simulink model "oving2e"  (R2020b)
settings: Solver=VariableStepAuto  StartTime=0.0  StopTime=10.0  RelTol=1e-3
values from neighbouring files (symbols this model uses):
  K = 1    [oving2script.m]
  l = 1    [Oving2Var.mat]    (also in oving2script.m)
  T = 1    [Oving2Var.mat]    (also in oving2script.m)
  y_0 = 0    [oving2script.m]
undefined symbols (not defined in the file or in its folder): K_i, K_p, r_0
settings Model: Creator=crezl  LastModifiedBy=crezl

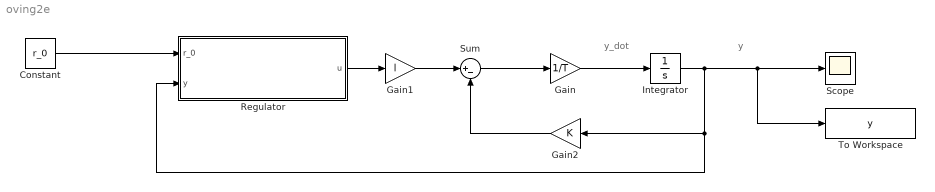
== system oving2e ==
  note: y_dot
  note: y
  Constant : Constant  Value=r_0
  Gain : Gain  Gain=1/T
  Gain1 : Gain  Gain=l
  Gain2 : Gain  Gain=K
  Integrator : Integrator  InitialCondition=y_0
  Regulator : Subsystem
  Scope : Scope
  Sum : Sum  Inputs=|+-
  To Workspace : ToWorkspace  VariableName=y  SaveFormat=Timeseries  SampleTime=-1
  wires:
  Gain/1 -> Integrator/1
  Gain2/1 -> Sum/2
  Sum/1 -> Gain/1
  Gain1/1 -> Sum/1
  Integrator/1 -> Regulator/2(y), Gain2/1, To Workspace/1, Scope/1
  Constant/1 -> Regulator/1(r_0)
  Regulator/1(u) -> Gain1/1

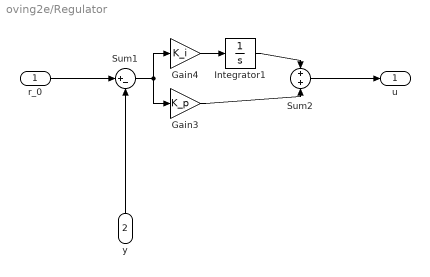
== system oving2e/Regulator ==
  r_0 : Inport
  y : Inport  Port=2
  Gain3 : Gain  Gain=K_p
  Gain4 : Gain  Gain=K_i
  Integrator1 : Integrator
  Sum1 : Sum  Inputs=|+-
  Sum2 : Sum  Inputs=+|+
  u : Outport
  wires:
  Sum1/1 -> Gain3/1, Gain4/1
  Gain4/1 -> Integrator1/1
  Integrator1/1 -> Sum2/1
  r_0/1 -> Sum1/1
  y/1 -> Sum1/2
  Sum2/1 -> u/1
  Gain3/1 -> Sum2/2
